simulink model "verify_Condensing_Boiler_CONF_mdl"  (R2016b)
settings: Solver=ode45  StartTime=0  StopTime=1800  MaxStep=10  RelTol=1e-3  EnableMultiTasking=on
undefined symbols (not defined in the file or in its folder): path_carnot
libraries: carnot x3, simulink x1
settings Model: Creator=drhf  LastModifiedBy=drhf
settings DataIOCC: SaveFormat=Array  SignalLoggingSaveFormat=ModelDataLogs
settings OptimizationCC: ExpressionDepthLimit=2147483647  LifeSpan=inf
settings DebuggingCC: UnderspecifiedInitializationDetection=Classic  MergeDetectMultiDrivingBlocksExec=none  SolverPrmCheckMsg=warning  FcnCallInpInsideContextMsg=warning  StateNameClashWarn=warning  SFUnexpectedBacktrackingDiag=warning  SFNoUnconditionalDefaultTransitionDiag=warning  SFExecutionAtInitializationDiag=none
settings HardwareCC: ProdBitPerPointer=32  ProdBitPerSizeT=32  ProdBitPerPtrDiffT=32  ProdLargestAtomicFloat=None  ProdIntDivRoundTo=Undefined  ProdEndianess=Unspecified  ProdWordSize=32  ProdHWDeviceType=32-bit Generic
settings ModelReferenceCC: PropagateSignalLabelsOutOfModel=off
settings GRTTargetCC: TargetLangStandard=C89/C90 (ANSI)  GeneratePreprocessorConditionals=Disable all  CombineOutputUpdateFcns=off  GRTInterface=on
settings ConfigComp: CovMetricSettings=dw  CovHtmlReporting=on  CovSaveCumulativeToWorkspaceVar=on  CovSaveSingleToWorkspaceVar=on  CovExternalEMLEnable=off

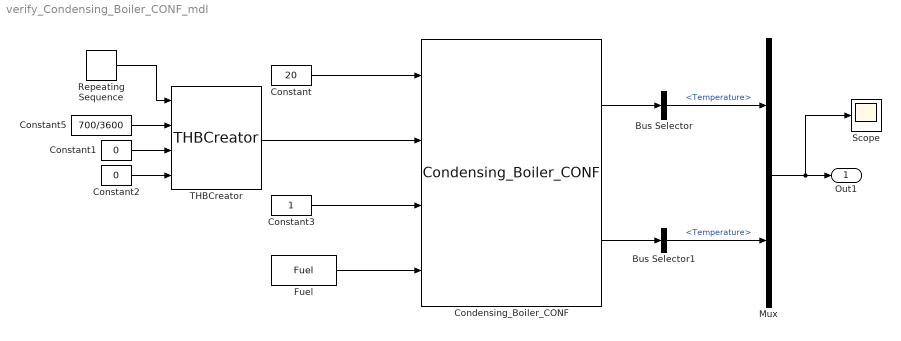
== system verify_Condensing_Boiler_CONF_mdl ==
  Bus Selector : BusSelector  OutputSignals=Temperature
  Bus Selector1 : BusSelector  OutputSignals=THBin.Temperature
  Condensing_Boiler_CONF : carnot/Source/Boiler/Condensing_Boiler_CONF  Tini=20  PathName=fullfile(path_carnot('libsl'), 'Source','Boiler','Condensing_Boiler_CONF','parameter_set')  FileName='DefaultCondensingBoiler.mat'  userPath=off  userParam=off  Pgas=20000  HeatLoss=2.5  Volume=0.0035  ElectricPower=[50 200]  TableRelativePower=[0.1 1]  whichTforEfficiency=mean of inlet and outlet temperature  TableData=[1 1;1 1]  TableTemperatures=[10 90]  relQdotMin=0.1  dplin=10  dpqua=100  Nodes=3
  Constant : Constant  Value=20
  Constant1 : Constant  Value=0
  Constant2 : Constant  Value=0
  Constant3 : Constant
  Constant5 : Constant  Value=700/3600
  Fuel : carnot/Source/Energy/Fuel  ft=1  t=20  ls=3.5  p=1.013e5  h_values=[5.14e7 5.69e7]  tc=45  price=1  mass=[0.33 0.67 0 0 0 0]
  Mux : Mux  Inputs=2
  Repeating Sequence : simulink/Sources/Repeating Sequence  rep_seq_t="[0 200  1500 1801]"  rep_seq_y=[30 30 65 65]
  Scope : Scope
  THBCreator : carnot/Basic/Hydraulics/THBCreator  Inport_ID=off  Inport_T=on  Inport_mdot=on  Inport_p=off  Inport_type=off  Inport_mix=off  Inport_mix2=on  Inport_mix3=on  Inport_d=off  Inport_c=off  Inport_l=off  Inport_q=off  Inport_LH=off  Inport_H=off  ID=20001  T=30  mdot=0  p=2e5  FluidType=1  FluidMix=0  FluidMix2=0  FluidMix3=0  d=0.02  c=0  l=0  q=0  LH=0  H=0  Annotation_ID=off  Annotation_T=off  Annotation_mdot=off  Annotation_p=off  Annotation_type=off  Annotation_mix=off  Annotation_mix2=off  Annotation_mix3=off  Annotation_d=off  Annotation_c=off  Annotation_l=off  Annotation_q=off  Annotation_LH=off  Annotation_H=off
  Out1 : Outport
  wires:
  Mux/1 -> Scope/1, Out1/1
  Condensing_Boiler_CONF/1 -> Bus Selector/1
  Condensing_Boiler_CONF/2 -> Bus Selector1/1
  Bus Selector/1 -> Mux/1  "<Temperature>"
  Bus Selector1/1 -> Mux/2  "<Temperature>"
  Constant5/1 -> THBCreator/2
  Repeating Sequence/1 -> THBCreator/1
  THBCreator/1 -> Condensing_Boiler_CONF/2
  Constant1/1 -> THBCreator/3
  Constant2/1 -> THBCreator/4
  Constant/1 -> Condensing_Boiler_CONF/1
  Constant3/1 -> Condensing_Boiler_CONF/3
  Fuel/1 -> Condensing_Boiler_CONF/4
